simulink model "modelado2"  (R2023a)
settings: Solver=VariableStepAuto  StartTime=0.0  StopTime=10.0  MaxStep=0.01  RelTol=1e-3
values from neighbouring files (symbols this model uses):
  g = 9.81    [modelado_2.m]
  l1 = 0.3    [modelado_2.m]
  l2 = 0.25    [modelado_2.m]
  m1 = 0.2    [modelado_2.m]
  m2 = 0.1    [modelado_2.m]

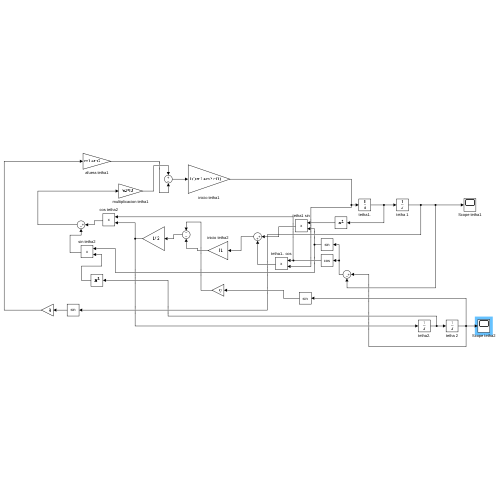
[thumbnail: Simulink's stored preview of the top-level diagram]
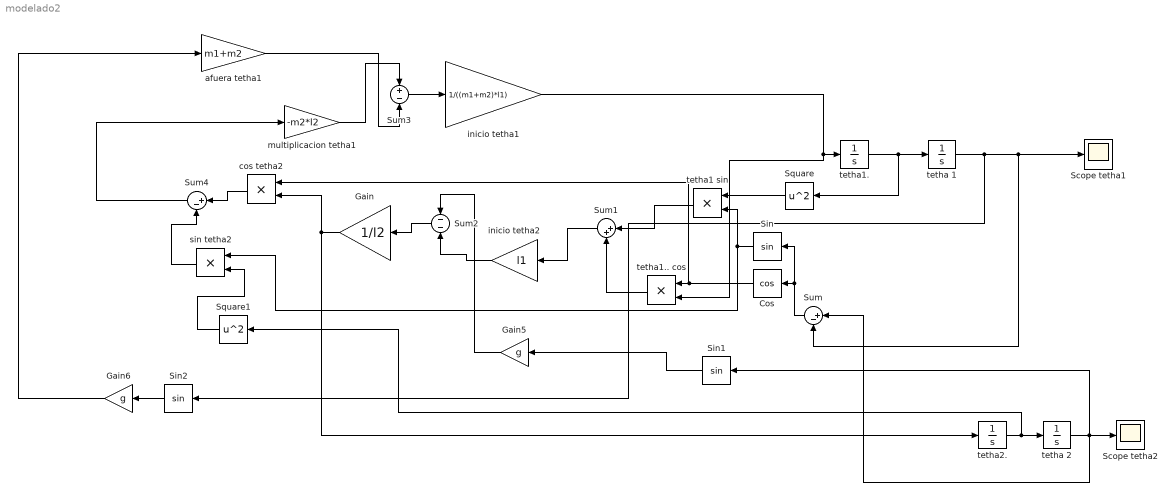
== system modelado2 ==
  Cos : Trigonometry  Operator=cos
  Gain : Gain  Gain=1/l2
  Gain5 : Gain  Gain=g
  Gain6 : Gain  Gain=g
  Scope tetha1 : Scope
  Scope tetha2 : Scope
  Sin : Trigonometry
  Sin1 : Trigonometry
  Sin2 : Trigonometry
  Square : Math  Operator=square
  Square1 : Math  Operator=square  SignedPower=on  RndMeth=Zero
  Sum : Sum  Inputs=|+-
  Sum1 : Sum  Inputs=|++
  Sum2 : Sum  Inputs=--
  Sum3 : Sum  Inputs=+-
  Sum4 : Sum  Inputs=|+-
  afuera tetha1 : Gain  Gain=m1+m2
  cos tetha2 : Product
  inicio tetha1 : Gain  Gain=1/((m1+m2)*l1)
  inicio tetha2 : Gain  Gain=l1
  multiplicacion tetha1 : Gain  Gain=-m2*l2
  sin tetha2 : Product
  tetha 1 : Integrator
  tetha 2 : Integrator  InitialCondition=(35*pi)/180
  tetha1 sin : Product
  tetha1. : Integrator
  tetha1.. cos : Product
  tetha2. : Integrator
  wires:
  tetha 1/1 -> Sin2/1, Sum/2, Scope tetha1/1
  tetha1./1 -> Square/1, tetha 1/1
  tetha2./1 -> Square1/1, tetha 2/1
  tetha 2/1 -> Sin1/1, Scope tetha2/1, Sum/1
  Sum/1 -> Sin/1, Cos/1
  Cos/1 -> cos tetha2/1, tetha1.. cos/1
  Square/1 -> tetha1 sin/1
  tetha1 sin/1 -> Sum1/1
  tetha1.. cos/1 -> Sum1/2
  Sum1/1 -> inicio tetha2/1
  inicio tetha2/1 -> Sum2/2
  Sin/1 -> tetha1 sin/2, sin tetha2/1
  Sum2/1 -> Gain/1
  Gain/1 -> cos tetha2/2, tetha2./1
  inicio tetha1/1 -> tetha1.. cos/2, tetha1./1
  Sum3/1 -> inicio tetha1/1
  cos tetha2/1 -> Sum4/1
  Square1/1 -> sin tetha2/2
  sin tetha2/1 -> Sum4/2
  Sum4/1 -> multiplicacion tetha1/1
  Gain6/1 -> afuera tetha1/1
  multiplicacion tetha1/1 -> Sum3/1
  afuera tetha1/1 -> Sum3/2
  Sin1/1 -> Gain5/1
  Gain5/1 -> Sum2/1
  Sin2/1 -> Gain6/1
